simulink model "w1p3"  (R2020b)
settings: Solver=VariableStepAuto  StartTime=0.0  StopTime=10.0  MaxStep=0.0001  RelTol=1e-3
settings Model: Creator=family  LastModifiedBy=family

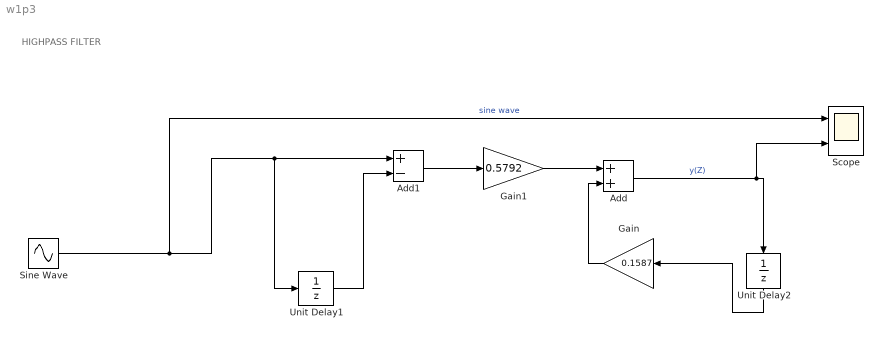
== system w1p3 ==
  note: HIGHPASS FILTER
  Add : Sum
  Add1 : Sum  Inputs=+-
  Gain : Gain  Gain=0.1587
  Gain1 : Gain  Gain=0.5792
  Scope : Scope  NumInputPorts=2
  Sine Wave : Sin  Frequency=500  SampleTime=0
  Unit Delay1 : UnitDelay  SampleTime=-1  HasFrameUpgradeWarning=on
  Unit Delay2 : UnitDelay  SampleTime=-1  HasFrameUpgradeWarning=on
  wires:
  Unit Delay1/1 -> Add1/2
  Add1/1 -> Gain1/1
  Gain1/1 -> Add/1
  Gain/1 -> Add/2
  Unit Delay2/1 -> Gain/1
  Add/1 -> Scope/2, Unit Delay2/1  "y(Z)"
  Sine Wave/1 -> Scope/1, Add1/1, Unit Delay1/1  "sine wave"
